simulink model "siavash_walking_o"  (R2015a)
settings: Solver=FixedStepDiscrete  StartTime=0.0  StopTime=inf  FixedStep=sample_time  RelTol=1e-3
StartFcn:
  | tg.sampletime = correctedSampleTime;
settings Model: SimulationMode=external  CovSFcnEnable=off  Creator=wmartin  LastModifiedBy=drl
settings SolverCC: EnableConcurrentExecution=on
settings DataIOCC: LimitDataPoints=off  MaxDataPoints=1e7  SaveFormat=StructureWithTime  SignalLogging=off  DSMLogging=off
settings OptimizationCC: BlockReduction=off  OptimizeBlockIOStorage=off  BufferReuse=off  GlobalBufferReuse=off  ExpressionFolding=off  ExpressionDepthLimit=2147483647  LocalBlockOutputs=off  SimCompilerOptimization=on
settings DebuggingCC: UnderspecifiedInitializationDetection=Classic  MergeDetectMultiDrivingBlocksExec=none  SolverPrmCheckMsg=warning  StateNameClashWarn=warning
settings HardwareCC: ProdIntDivRoundTo=Zero  ProdEndianess=LittleEndian  ProdLongLongMode=on  ProdHWDeviceType=Generic->32-bit x86 compatible
settings ModelReferenceCC: UpdateModelReferenceTargets=IfOutOfDate  ModelReferenceNumInstancesAllowed=Single  ModelReferenceMinAlgLoopOccurrences=on
settings RTWCC: SystemTargetFile=slrt.tlc  TemplateMakefile=slrt_default_tmf  Description=Simulink Real-Time  RTWVerbose=off  RTWCompilerOptimization=on
settings CodeAppCC: MaxIdLength=256
settings SimulinkRealTimeCC: GeneratePreprocessorConditionals=Disable all  RL32LogBufSizeModifier=1e8

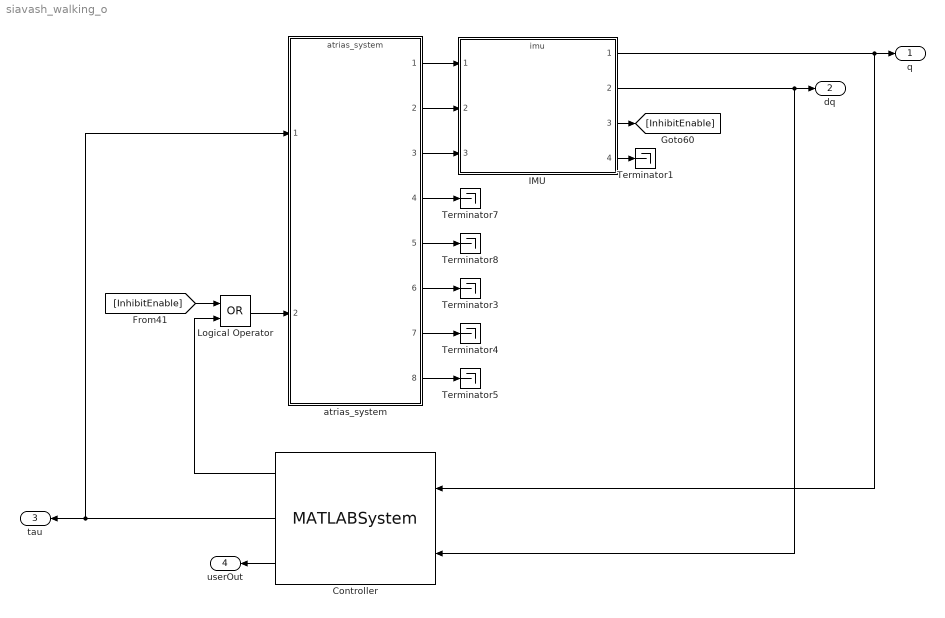
== system siavash_walking_o ==
  Controller : MATLABSystem  System=siavash_walkNrunNhop  isTimeTrig=on  isForceTrig=on  sT=[1.1 1.02 1.1 0.88]  k_fp_h_v=0.23  k_fp_l_v=0.26  k_fp_h_e=.07  k_fp_l_e=0.05  T0=0.35  k_time=0.015  kDx=.1  kDy=0  xss=0  yss=0.18  ys0v=0  kv_yss=0.015  kv_h=0.005  kv_l=0.005  lret=0.2  l0=0.9  kp_leg=3000  kd_leg=120  kp_hip=2000  kd_hip=75  legRetPerc=40  k_Energy=0.021  ll_dev=0.13  k_hop=1  mu_s=.5  isAngular=false  isYawTraj=true  torso_ff=1  isSim=off  ps3Axes=[0 0 0 0]  ps3Buttons=zeros([1 17])  u_lim=600  SimulateUsing=Code generation
      mask Type: siavash_walkNrunNhop
      mask Display:
      | disp('siavash_walkNrunNhop');
      | port_label('input',1,'q');
      | port_label('input',2,'dq');
      | port_label('output',1,'eStop');
      | port_label('output',2,'u');
      | port_label('output',3,'userOut');
  IMU : ModelReference  ModelNameDialog=imu  SimulationMode=Normal  ModelReferenceVersion=1.2453  CopyOfModelName=imu  DefaultDataLogging=on
  Logical Operator : Logic  Operator=OR  AllPortsSameDT=off  OutDataTypeStr=boolean
  Terminator{1,3..5,7..8} (6 alike) : Terminator
  atrias_system : ModelReference  ModelNameDialog=atrias_system  SimulationMode=Normal  ModelReferenceVersion=1.2776  CopyOfModelName=atrias_system  DefaultDataLogging=on
  q : Outport
  dq : Outport  Port=2
  tau : Outport  Port=3
  userOut : Outport  Port=4
  wires:
  atrias_system/4 -> Terminator7/1
  atrias_system/7 -> Terminator4/1
  atrias_system/6 -> Terminator3/1
  atrias_system/8 -> Terminator5/1
  Controller/2 -> tau/1, atrias_system/1
  IMU/3 -> [InhibitEnable]
  IMU/1 -> Controller/1, q/1
  IMU/2 -> dq/1, Controller/2
  atrias_system/1 -> IMU/1
  atrias_system/2 -> IMU/2
  atrias_system/3 -> IMU/3
  [InhibitEnable] -> Logical Operator/1
  Logical Operator/1 -> atrias_system/2
  Controller/1 -> Logical Operator/2
  Controller/3 -> userOut/1
  atrias_system/5 -> Terminator8/1
  IMU/4 -> Terminator1/1
